simulink model "ej2_2"  (R2023a)
settings: Solver=VariableStepAuto  StartTime=0.0  StopTime=30  RelTol=1e-3
values from neighbouring files (symbols this model uses):
  b = 8/3    (= 2.66666666667)    [ej2_2_script.m]
  r = 0.9    [ej2_2_script.m]
  s = 10    [ej2_2_script.m]
settings Model: Creator=erwinplanck  LastModifiedBy=erwinplanck

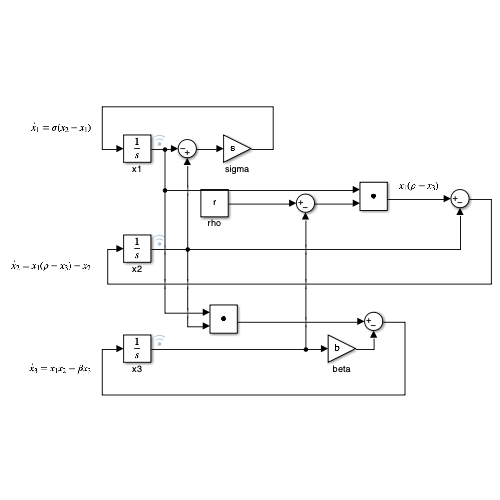
[thumbnail: Simulink's stored preview of the top-level diagram]
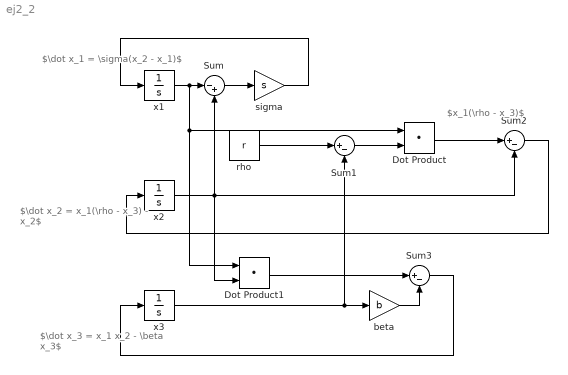
== system ej2_2 ==
  note: $x_1(\rho - x_3)$
  note: $\dot x_2 = x_1(\rho - x_3) - x_2$
  note: $\dot x_1 = \sigma(x_2 - x_1)$
  note: $\dot x_3 = x_1 x_2 - \beta x_3$
  Dot Product : DotProduct  OutDataTypeStr=Inherit: Inherit via internal rule
  Dot Product1 : DotProduct  OutDataTypeStr=Inherit: Inherit via internal rule
  Sum : Sum  Inputs=|-+
  Sum1 : Sum  Inputs=|+-
  Sum2 : Sum  Inputs=|+-
  Sum3 : Sum  Inputs=|+-
  beta : Gain  Gain=b
  rho : Constant  Value=r
  sigma : Gain  Gain=s
  x1 : Integrator  InitialCondition=1
  x2 : Integrator  InitialCondition=1
  x3 : Integrator  InitialCondition=1
  wires:
  x2/1 -> Sum2/2, Sum/2, Dot Product1/2
  x1/1 -> Dot Product1/1, Dot Product/1, Sum/1
  Sum/1 -> sigma/1
  sigma/1 -> x1/1
  rho/1 -> Sum1/1
  x3/1 -> beta/1, Sum1/2
  Sum1/1 -> Dot Product/2
  Dot Product/1 -> Sum2/1
  Sum2/1 -> x2/1
  Dot Product1/1 -> Sum3/1
  beta/1 -> Sum3/2
  Sum3/1 -> x3/1
